simulink model "wave2"  (R2016b)
settings: Solver=VariableStepAuto  StartTime=0.0  StopTime=40.0  RelTol=1e-3
libraries: simulink x2
settings Model: Creator=charAn  LastModifiedBy=charAn

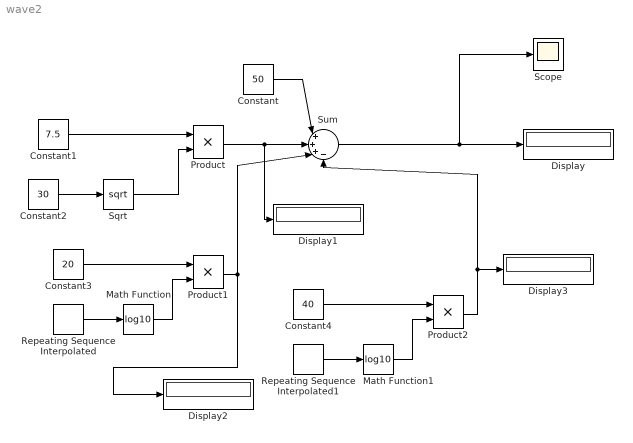
== system wave2 ==
  Constant : Constant  Value=50
  Constant1 : Constant  Value=7.5
  Constant2 : Constant  Value=30
  Constant3 : Constant  Value=20
  Constant4 : Constant  Value=40
  Display{,1..3} (4 alike) : Display
  Math Function : Math  Operator=log10  SaturateOnIntegerOverflow=on
  Math Function1 : Math  Operator=log10  SaturateOnIntegerOverflow=on
  Product : Product
  Product1 : Product
  Product2 : Product
  Repeating Sequence Interpolated : simulink/Sources/Repeating Sequence Interpolated  OutValues=[0 50 100 150 200]  TimeValues=[0 10 20 30 40 ]  LookUpMeth=Interpolation-Use End Values  tsamp=0.01  OutMin=[]  OutMax=[]  OutDataTypeStr=double  OutputDataTypeScalingMode=double  OutDataType=fixdt(0,8)  OutScaling=2^-10
  Repeating Sequence Interpolated1 : simulink/Sources/Repeating Sequence Interpolated  OutValues=[0.4 50.4 100.4 150.4 200.4]  TimeValues=[0 10 20 30 40 ]  LookUpMeth=Interpolation-Use End Values  tsamp=0.01  OutMin=[]  OutMax=[]  OutDataTypeStr=double  OutputDataTypeScalingMode=double  OutDataType=fixdt(0,8)  OutScaling=2^-10
  Scope : Scope
  Sqrt : Sqrt  SaturateOnIntegerOverflow=on
  Sum : Sum  Inputs=|+++-
  wires:
  Constant2/1 -> Sqrt/1
  Constant1/1 -> Product/1
  Sqrt/1 -> Product/2
  Product/1 -> Display1/1, Sum/2
  Constant/1 -> Sum/1
  Repeating Sequence Interpolated/1 -> Math Function/1
  Constant3/1 -> Product1/1
  Math Function/1 -> Product1/2
  Repeating Sequence Interpolated1/1 -> Math Function1/1
  Constant4/1 -> Product2/1
  Math Function1/1 -> Product2/2
  Product2/1 -> Display3/1, Sum/4
  Sum/1 -> Scope/1, Display/1
  Product1/1 -> Display2/1, Sum/3
